simulink model "new"  (R2020a)
settings: Solver=VariableStepAuto  StartTime=0.0  StopTime=10.0  RelTol=1e-3
settings Model: Creator=Marcus  LastModifiedBy=Marcus

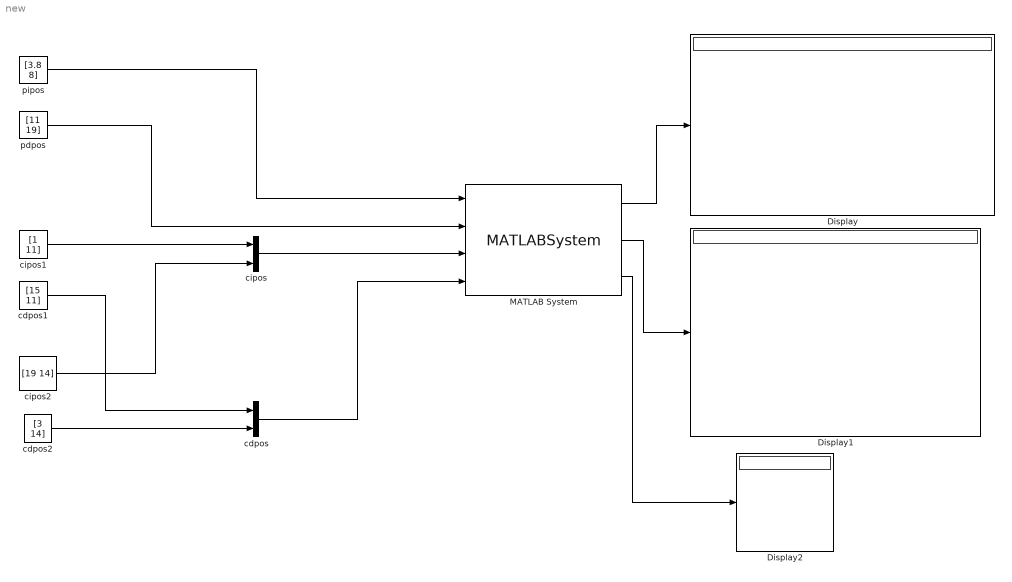
== system new ==
  Display : Display
  Display1 : Display
  Display2 : Display
  MATLAB System : MATLABSystem  System=trajPlanner2  SimulateUsing=Interpreted execution
      mask Type: trajPlanner2
      mask Display:
      | disp('trajPlanner2');
      | port_label('input',1,'pipos');
      | port_label('input',2,'pdpos');
      | port_label('input',3,'cipos');
      | port_label('input',4,'cdpos');
      | port_label('output',1,'ptraj');
      | port_label('output',2,'ctraj');
      | port_label('output',3,'coll');
  "cdpos " : Concatenate
  cdpos1 : Constant  Value=[15 11]
  cdpos2 : Constant  Value=[3 14]
  cipos : Concatenate
  cipos1 : Constant  Value=[1 11]
  cipos2 : Constant  Value=[19 14]
  pdpos : Constant  Value=[11 19]
  pipos : Constant  Value=[3.8 8]
  wires:
  cipos1/1 -> cipos/1
  cipos2/1 -> cipos/2
  cdpos2/1 -> "cdpos "/2
  cdpos1/1 -> "cdpos "/1
  cipos/1 -> MATLAB System/3
  "cdpos "/1 -> MATLAB System/4
  pipos/1 -> MATLAB System/1
  pdpos/1 -> MATLAB System/2
  MATLAB System/3 -> Display2/1
  MATLAB System/2 -> Display1/1
  MATLAB System/1 -> Display/1
